simulink model "FOC_DQ0"  (R2022b)
settings: Solver=FixedStepAuto  StartTime=0.0  StopTime=20
values from neighbouring files (symbols this model uses):
  battery = struct()    [FOC_DQ0_parameters.m]
  motor = struct()    [FOC_DQ0_parameters.m]
libraries: simulink_extras x3, simulink x1
settings Model: Creator=dwegg  LastModifiedBy=dwegg
settings SolverCC: MaxConsecutiveZCs=auto  AlgebraicLoopSolver=TrustRegion
settings OptimizationCC: OptimizeBlockIOStorage=off  OptimizeDataStoreBuffers=off  BusAssignmentInplaceUpdate=off
settings DebuggingCC: UnconnectedInputMsg=warning  UnconnectedOutputMsg=warning  UnconnectedLineMsg=warning  SFUnexpectedBacktrackingDiag=warning  SFNoUnconditionalDefaultTransitionDiag=warning  SFMachineParentedDataDiag=warning
settings ModelReferenceCC: EnableRefExpFcnMdlSchedulingChecks=on
settings RTWCC: GenCodeOnly=on  GenerateReport=on  BuildConfiguration=Debug  LaunchReport=on  DLArmComputeVersion=19.05
settings CodeAppCC: ForceParamTrailComments=on  MATLABSourceComments=on  EnableCustomComments=on
settings GRTTargetCC: CombineSignalStateStructs=on  SupportVariableSizeSignals=on  MultiInstanceErrorCode=Warning

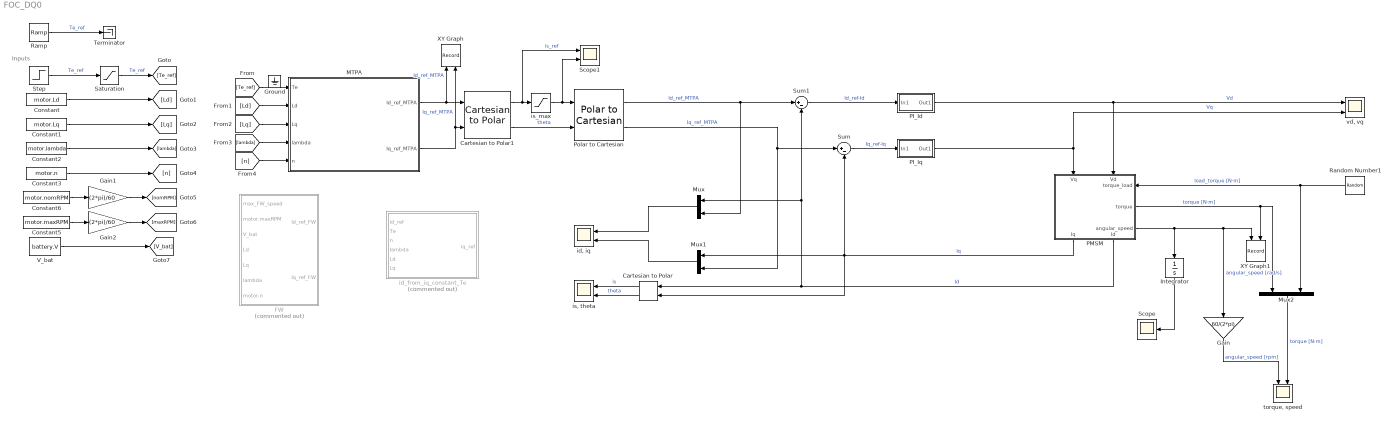
== system FOC_DQ0 ==
  note: Inputs
  Cartesian to Polar : simulink_extras/Transformations/Cartesian to Polar
  Cartesian to Polar1 : simulink_extras/Transformations/Cartesian to Polar
  Constant : Constant  Value=motor.Ld
  Constant1 : Constant  Value=motor.Lq
  Constant2 : Constant  Value=motor.lambda
  Constant3 : Constant  Value=motor.n
  Constant5 : Constant  Value=motor.maxRPM
  Constant6 : Constant  Value=motor.nomRPM
  FW : Subsystem  Commented=on
  Gain : Gain  Gain=60/(2*pi)
  Gain1 : Gain  Gain=(2*pi)/60
  Gain2 : Gain  Gain=(2*pi)/60
  Integrator : Integrator  UpperSaturationLimit=2*pi  LowerSaturationLimit=0  WrapState=on
  MTPA : Subsystem
  Mux : Mux  Inputs=2
  Mux1 : Mux  Inputs=2
  Mux2 : Mux  Inputs=2
  PI_Id : Subsystem
  PI_Iq : Subsystem
  PMSM : Subsystem
      settings: PortSchema="{\"entries\":[{\"content\":{\"sides\":[{\"content\":{\"connectorIds\":[\"In1\",\"In2\"]},\"type\":\"ConnectorPlacement.EquallySpacedRectSide\",\"uuid\":\"acf6d0e8-5fcc-4ac9-9f91-0b0686f5c890\"},{\"content\":{\"connectorIds\":[\"Out1\",\"Out2\"],\"side\":\"RIGHT\"},\"type\":\"ConnectorPlacement.EquallySpacedRectSide\",\"uuid\":\"62f3436c-1459-412f-a025-ace7c361d3d0\"},{\"content\":{\"connectorIds\":[\"In3\",\"Out3\",\"Out4\"],\"side\":\"TOP\"},\"type\":\"ConnectorPlacement.EquallySpacedRectSide\",\"uuid\":\"813607d4-1b75-442b-b64c-87c67b317e31\"},{\"content\":{\"connectorIds\":[],\"side\":\"HIDDEN\"},\"type\":\"ConnectorPlacement.EquallySpacedRectSide\",\"uuid\":\"b791fad5-6496-44b1-9d55-edef34be28ea\"}]},\"type\":\"ConnectorPlacement.EquallySpacedConnector\",\"uuid\":\"ea6ad5c4-a0c3-44bf-8a7e-ca4afd038dbb\"}],\"packageUris\":[\"http://schema.mathworks.com/mf0/Connector/R2020b\"],\"version\":\"1.0\"}"
      mask Display: image('$imagefile'); % Use "Edit Image" on toolstrip to change.
  Polar to Cartesian : simulink_extras/Transformations/Polar to Cartesian
  Ramp : simulink/Sources/Ramp  slope=-5  start=1  InitialOutput=40
  Random Number1 : RandomNumber  Variance=0  SampleTime=0.1
  Saturation : Saturate  UpperLimit=40  LowerLimit=-40
  Scope : Scope
  Scope1 : Scope  NumInputPorts=2
  Step : Step  After=26  SampleTime=0
  Sum : Sum  Inputs=|+-
  Sum1 : Sum  Inputs=|+-
  Terminator : Terminator
  V_bat : Constant  Value=battery.V
  XY Graph : Record  FileSettingsInternal="{\"entries\":[{\"content\":{\"excelSettings\":{\"content\":{},\"type\":\"Streamout.ExcelSettings\"}},\"type\":\"Streamout.FileSettingStorage\",\"uuid\":\"a65b38da-4a6e-42be-b919-12943431f1e8\"}],\"packageUris\":[\"http://schema.mathworks.com/mf0/streamout_blocks/R2020a\"],\"version\":\"1.0\"}"  Layout=[1 1]  SignalsInternal="{\"entries\":[{\"content\":{\"signals\":[{\"content\":{\"blockPath\":[\"FOC_DQ0/XY Graph\"],\"channel\":[],\"dimensions\":[1],\"domain\":\"FOC_DQ0/XY Graph\",\"lineColor\":\"#b746ff\",\"plots\":[1],\"port\":1,\"sid\":[\"\"],\"signalID\":27,\"signalName\":\"Id_ref_MTPA\"},\"type\":\"RecordBlkView.Signal\",\"uuid\":\"71ded6d7-b5de-456d-a39b-39459f0f97cd\"},{\"content\":{\"blockPath\":[\"FOC_DQ0/XY Graph\"],\"channel\":[],\"dimensions\":[1],\"domain\":\"FOC_DQ0/XY Graph\",\"lineColor\":\"#ff13a6\",\"plots\":[1],\"port\":2,\"sid\":[\"\"],\"signalID\":31,\"signalName\":\"Iq_ref_MTPA\"},\"type\":\"RecordBlkView.Signal\",\"uuid\":\"91d96bc1-a89e-499f-a0a8-186399ce3372\"}]},\"type\":\"RecordBlkView.InputSignals\",\"uuid\":\"76abfc2d-da4e-48c8-a2e1-e55e58ffb88b\"}],\"packageUris\":[\"http://schema.mathworks.com/mf0/streamout_blocks/R2020a\"],\"version\":\"1.0\"}"  VisualizationBindings="{\"xyplotplugin\":{\"info\":[{\"series\":[{\"bindingParametersList\":[{\"parameter\":\"X-Axis\",\"signalID\":27,\"signalName\":\"Id_ref_MTPA\"},{\"parameter\":\"Y-Axis\",\"signalID\":31,\"signalName\":\"Iq_ref_MTPA\"}],\"seriesID\":34336}],\"subplotID\":1}]}}"  CompatibilityTag=XY
  XY Graph1 : Record  FileSettingsInternal="{\"entries\":[{\"content\":{\"excelSettings\":{\"content\":{},\"type\":\"Streamout.ExcelSettings\"}},\"type\":\"Streamout.FileSettingStorage\",\"uuid\":\"c1a863bd-84bc-484d-b47a-9520c9f9713e\"}],\"packageUris\":[\"http://schema.mathworks.com/mf0/streamout_blocks/R2020a\"],\"version\":\"1.0\"}"  Layout=[1 1]  SignalsInternal="{\"entries\":[{\"content\":{\"signals\":[{\"content\":{\"blockPath\":[\"FOC_DQ0/XY Graph1\"],\"channel\":[],\"dimensions\":[1],\"domain\":\"FOC_DQ0/XY Graph1\",\"lineColor\":\"#a2142f\",\"plots\":[1],\"port\":1,\"sid\":[\"\"],\"signalID\":35,\"signalName\":\"angular_speed [rad/s]\"},\"type\":\"RecordBlkView.Signal\",\"uuid\":\"696599aa-ddef-40f7-9026-a933a86ecc6f\"},{\"content\":{\"blockPath\":[\"FOC_DQ0/XY Graph1\"],\"channel\":[],\"dimensions\":[1],\"domain\":\"FOC_DQ0/XY Graph1\",\"lineColor\":\"#139fff\",\"plots\":[1],\"port\":2,\"sid\":[\"\"],\"signalID\":39,\"signalName\":\"torque [N·m]\"},\"type\":\"RecordBlkView.Signal\",\"uuid\":\"06b63f20-2c7a-4cdb-9373-f78a38729ebe\"}]},\"type\":\"RecordBlkView.InputSignals\",\"uuid\":\"cbe1f972-30dc-467d-b6c0-ab8105ad27ef\"}],\"packageUris\":[\"http://schema.mathworks.com/mf0/streamout_blocks/R2020a\"],\"version\":\"1.0\"}"  VisualizationBindings="{\"xyplotplugin\":{\"info\":[{\"series\":[{\"bindingParametersList\":[{\"parameter\":\"X-Axis\",\"signalID\":35,\"signalName\":\"angular_speed [rad\\/s]\"},{\"parameter\":\"Y-Axis\",\"signalID\":39,\"signalName\":\"torque [N·m]\"}],\"seriesID\":51202}],\"subplotID\":1}]}}"  CompatibilityTag=XY
  "id, iq" : Scope  NumInputPorts=2
  id_from_iq_constant_Te : MATLAB Function  Commented=on  TreatAsAtomicUnit=on
  "is, theta" : Scope  NumInputPorts=2
  is_max : Saturate  UpperLimit=motor.I_max  LowerLimit=-motor.I_max
  "torque, speed" : Scope  NumInputPorts=2
  "vd, vq" : Scope  NumInputPorts=2
  Ground : Ground  IOType=siggen
  wires:
  Random Number1/1 -> Mux2/2, PMSM/3(torque_load)  "load_torque [N·m]"
  PI_Iq/1(Out1) -> "vd, vq"/2, PMSM/2(Vq)  "Vq"
  PI_Id/1(Out1) -> PMSM/1(Vd), "vd, vq"/1  "Vd"
  Sum/1 -> PI_Iq/1(In1)  "Iq_ref-Iq"
  Sum1/1 -> PI_Id/1(In1)  "Id_ref-Id"
  PMSM/1(Id) -> Mux/1, Sum1/2, Cartesian to Polar/1  "Id"
  Mux/1 -> "id, iq"/1
  Mux1/1 -> "id, iq"/2
  PMSM/3(torque) -> XY Graph1/2, Mux2/1  "torque [N·m]"
  PMSM/4(angular_speed) -> Integrator/1, XY Graph1/1, Gain/1  "angular_speed [rad/s]"
  Gain/1 -> "torque, speed"/1  "angular_speed [rpm]"
  Mux2/1 -> "torque, speed"/2  "torque [N·m]"
  Saturation/1 -> [Te_ref]  "Te_ref"
  Polar to Cartesian/1 -> Mux/2, Sum1/1  "Id_ref_MTPA"
  Polar to Cartesian/2 -> Sum/1, Mux1/2  "Iq_ref_MTPA"
  Constant6/1 -> Gain1/1
  Cartesian to Polar/1 -> "is, theta"/1  "is"
  Cartesian to Polar/2 -> "is, theta"/2  "theta"
  Constant/1 -> [Ld]
  Constant1/1 -> [Lq]
  Constant2/1 -> [lambda]
  Constant3/1 -> [n]
  Gain1/1 -> [nomRPM]
  Constant5/1 -> Gain2/1
  Gain2/1 -> [maxRPM]
  V_bat/1 -> [V_bat]
  [Te_ref] -> MTPA/1(Te)
  [Ld] -> MTPA/2(Ld)
  [Lq] -> MTPA/3(Lq)
  [lambda] -> MTPA/4(lambda)
  [n] -> MTPA/5(n)
  Step/1 -> Saturation/1  "Te_ref"
  MTPA/1(Id_ref_MTPA) -> XY Graph/1, Cartesian to Polar1/1  "Id_ref_MTPA"
  MTPA/2(Iq_ref_MTPA) -> XY Graph/2, Cartesian to Polar1/2  "Iq_ref_MTPA"
  Cartesian to Polar1/2 -> Polar to Cartesian/2  "theta"
  Cartesian to Polar1/1 -> Scope1/1, is_max/1  "is_ref"
  is_max/1 -> Scope1/2, Polar to Cartesian/1
  PMSM/2(Iq) -> Mux1/1, Cartesian to Polar/2, Sum/2  "Iq"
  Integrator/1 -> Scope/1
  Ramp/1 -> Terminator/1  "Te_ref"

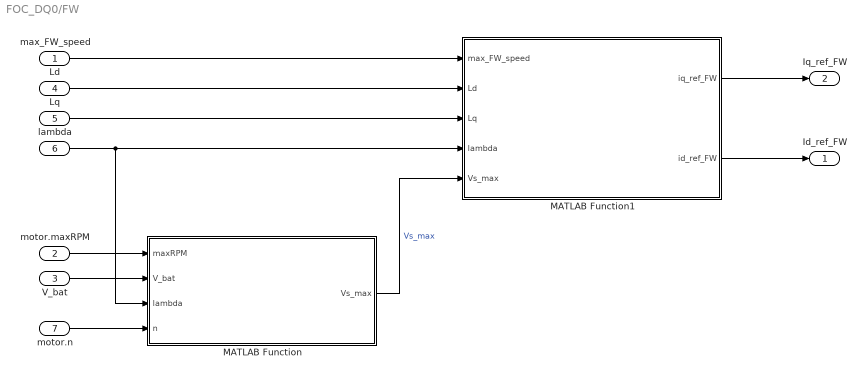
== system FOC_DQ0/FW ==
  max_FW_speed : Inport
  motor.maxRPM : Inport  Port=2
  V_bat : Inport  Port=3
  Ld : Inport  Port=4
  Lq : Inport  Port=5
  lambda : Inport  Port=6
  motor.n : Inport  Port=7
  MATLAB Function : MATLAB Function  TreatAsAtomicUnit=on
  MATLAB Function1 : MATLAB Function  TreatAsAtomicUnit=on
  Id_ref_FW : Outport
  Iq_ref_FW : Outport  Port=2
  wires:
  motor.maxRPM/1 -> MATLAB Function/1(maxRPM)
  V_bat/1 -> MATLAB Function/2(V_bat)
  MATLAB Function/1(Vs_max) -> MATLAB Function1/5(Vs_max)  "Vs_max"
  max_FW_speed/1 -> MATLAB Function1/1(max_FW_speed)
  Ld/1 -> MATLAB Function1/2(Ld)
  Lq/1 -> MATLAB Function1/3(Lq)
  lambda/1 -> MATLAB Function/3(lambda), MATLAB Function1/4(lambda)
  MATLAB Function1/1(iq_ref_FW) -> Iq_ref_FW/1
  MATLAB Function1/2(id_ref_FW) -> Id_ref_FW/1
  motor.n/1 -> MATLAB Function/4(n)

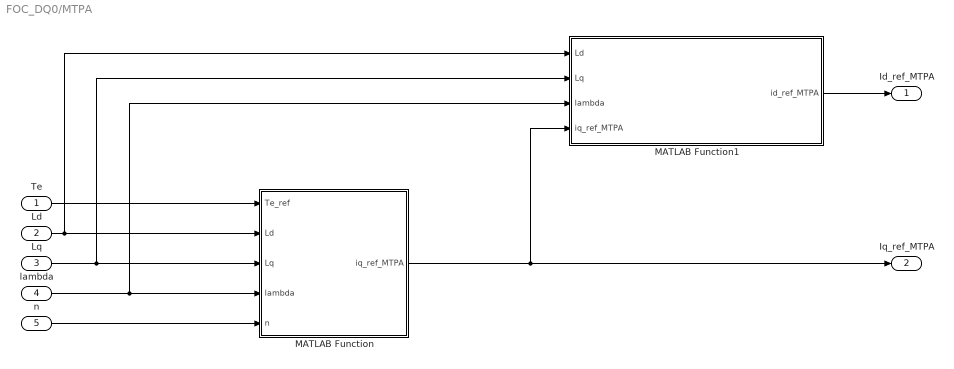
== system FOC_DQ0/MTPA ==
  Te : Inport
  Ld : Inport  Port=2
  Lq : Inport  Port=3
  lambda : Inport  Port=4
  n : Inport  Port=5
  MATLAB Function : MATLAB Function  TreatAsAtomicUnit=on
  MATLAB Function1 : MATLAB Function  TreatAsAtomicUnit=on
  Id_ref_MTPA : Outport
  Iq_ref_MTPA : Outport  Port=2
  wires:
  MATLAB Function/1(iq_ref_MTPA) -> MATLAB Function1/4(iq_ref_MTPA), Iq_ref_MTPA/1
  Te/1 -> MATLAB Function/1(Te_ref)
  Ld/1 -> MATLAB Function/2(Ld), MATLAB Function1/1(Ld)
  Lq/1 -> MATLAB Function1/2(Lq), MATLAB Function/3(Lq)
  lambda/1 -> MATLAB Function1/3(lambda), MATLAB Function/4(lambda)
  n/1 -> MATLAB Function/5(n)
  MATLAB Function1/1(id_ref_MTPA) -> Id_ref_MTPA/1

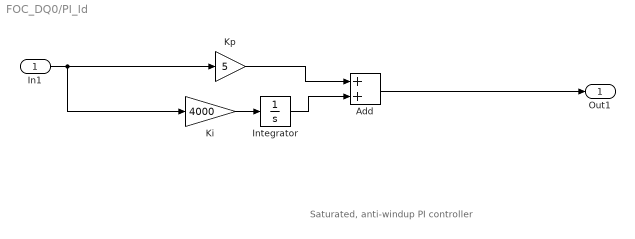
== system FOC_DQ0/PI_Id ==
  note: Saturated, anti-windup PI controller
  In1 : Inport
  Add : Sum
  Integrator : Integrator
  Ki : Gain  Gain=4000
  Kp : Gain  Gain=5
  Out1 : Outport
  wires:
  In1/1 -> Ki/1, Kp/1
  Kp/1 -> Add/1
  Integrator/1 -> Add/2
  Ki/1 -> Integrator/1
  Add/1 -> Out1/1

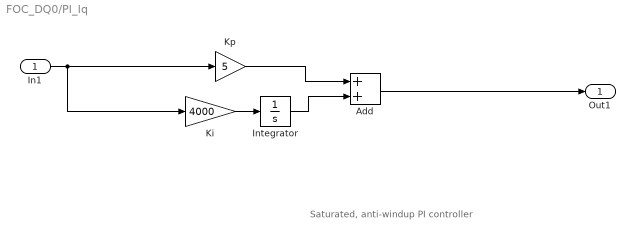
== system FOC_DQ0/PI_Iq ==
  note: Saturated, anti-windup PI controller
  In1 : Inport
  Add : Sum
  Integrator : Integrator
  Ki : Gain  Gain=4000
  Kp : Gain  Gain=5
  Out1 : Outport
  wires:
  Ki/1 -> Integrator/1
  Integrator/1 -> Add/2
  Kp/1 -> Add/1
  Add/1 -> Out1/1
  In1/1 -> Ki/1, Kp/1

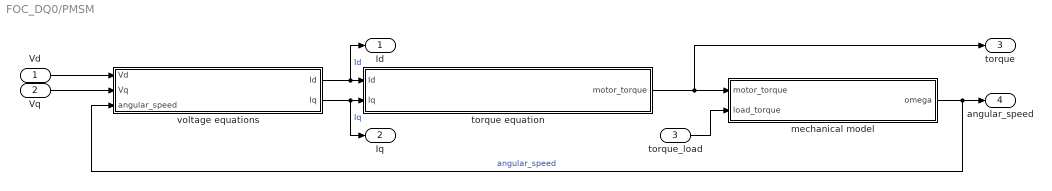
== system FOC_DQ0/PMSM ==
  Vd : Inport
  Vq : Inport  Port=2
  torque_load : Inport  Port=3
  mechanical model : Subsystem
      mask Display: image('$imagefile'); % Use "Edit Image" on toolstrip to change.
  torque equation : Subsystem
      mask Display: image('$imagefile'); % Use "Edit Image" on toolstrip to change.
  voltage equations : Subsystem
      mask Display: image('$imagefile'); % Use "Edit Image" on toolstrip to change.
  Id : Outport
  Iq : Outport  Port=2
  torque : Outport  Port=3
  angular_speed : Outport  Port=4
  wires:
  torque equation/1(motor_torque) -> torque/1, mechanical model/1(motor_torque)
  torque_load/1 -> mechanical model/2(load_torque)
  mechanical model/1(omega) -> angular_speed/1, voltage equations/3(angular_speed)  "angular_speed"
  voltage equations/2(Iq) -> Iq/1, torque equation/2(Iq)  "Iq"
  voltage equations/1(Id) -> Id/1, torque equation/1(Id)  "Id"
  Vd/1 -> voltage equations/1(Vd)
  Vq/1 -> voltage equations/2(Vq)

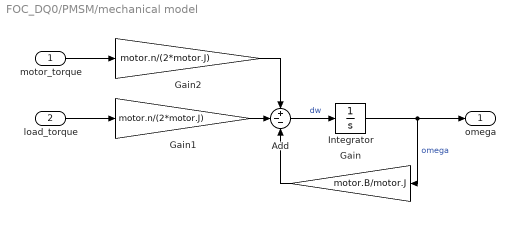
== system FOC_DQ0/PMSM/mechanical model ==
  motor_torque : Inport
  load_torque : Inport  Port=2
  Add : Sum  Inputs=+--
  Gain : Gain  Gain=motor.B/motor.J
  Gain1 : Gain  Gain=motor.n/(2*motor.J)
  Gain2 : Gain  Gain=motor.n/(2*motor.J)
  Integrator : Integrator
  omega : Outport
  wires:
  Gain1/1 -> Add/2
  Gain/1 -> Add/3
  Gain2/1 -> Add/1
  Add/1 -> Integrator/1  "dw"
  Integrator/1 -> omega/1, Gain/1  "omega"
  motor_torque/1 -> Gain2/1
  load_torque/1 -> Gain1/1

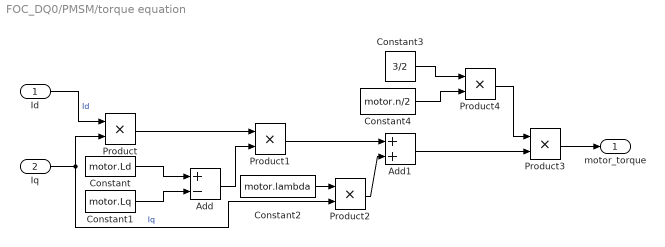
== system FOC_DQ0/PMSM/torque equation ==
  Id : Inport
  Iq : Inport  Port=2
  Add : Sum  Inputs=+-
  Add1 : Sum
  Constant : Constant  Value=motor.Ld
  Constant1 : Constant  Value=motor.Lq
  Constant2 : Constant  Value=motor.lambda
  Constant3 : Constant  Value=3/2
  Constant4 : Constant  Value=motor.n/2
  Product{,1..4} (5 alike) : Product
  motor_torque : Outport
  wires:
  Product1/1 -> Add1/1
  Add/1 -> Product1/2
  Constant4/1 -> Product4/2
  Constant2/1 -> Product2/1
  Add1/1 -> Product3/2
  Constant/1 -> Add/1
  Product/1 -> Product1/1
  Product4/1 -> Product3/1
  Constant3/1 -> Product4/1
  Product2/1 -> Add1/2
  Iq/1 -> Product/2, Product2/2  "Iq"
  Constant1/1 -> Add/2
  Product3/1 -> motor_torque/1
  Id/1 -> Product/1  "Id"

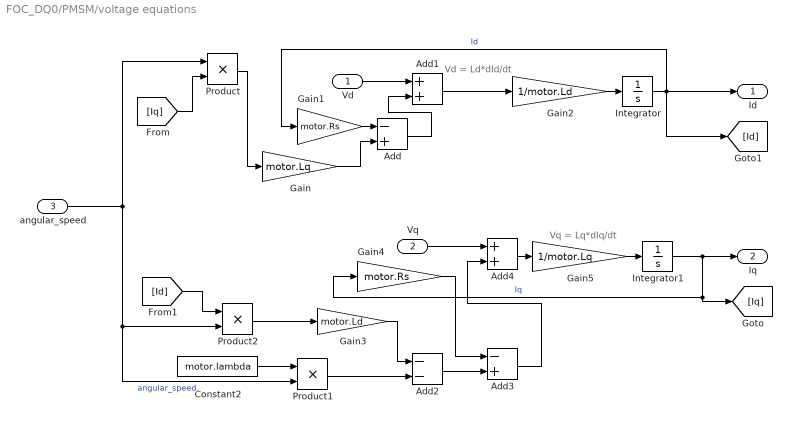
== system FOC_DQ0/PMSM/voltage equations ==
  note: Vd = Ld*dId/dt
  note: Vq = Lq*dIq/dt
  Vd : Inport
  Vq : Inport  Port=2
  angular_speed : Inport  Port=3
  Add : Sum  Inputs=-+
  Add1 : Sum
  Add2 : Sum  Inputs=--
  Add3 : Sum  Inputs=-+
  Add4 : Sum
  Constant2 : Constant  Value=motor.lambda
  Gain : Gain  Gain=motor.Lq
  Gain1 : Gain  Gain=motor.Rs
  Gain2 : Gain  Gain=1/motor.Ld
  Gain3 : Gain  Gain=motor.Ld
  Gain4 : Gain  Gain=motor.Rs
  Gain5 : Gain  Gain=1/motor.Lq
  Integrator : Integrator
  Integrator1 : Integrator
  Product : Product
  Product1 : Product
  Product2 : Product
  Id : Outport
  Iq : Outport  Port=2
  wires:
  angular_speed/1 -> Product2/2, Product1/2, Product/1  "angular_speed"
  Product/1 -> Gain/1
  Gain/1 -> Add/2
  Gain1/1 -> Add/1
  Integrator/1 -> Gain1/1, [Id], Id/1  "Id"
  Gain2/1 -> Integrator/1
  Add1/1 -> Gain2/1
  Add/1 -> Add1/2
  Vd/1 -> Add1/1
  Constant2/1 -> Product1/1
  Product2/1 -> Gain3/1
  Gain3/1 -> Add2/1
  Product1/1 -> Add2/2
  Add2/1 -> Add3/2
  Gain4/1 -> Add3/1
  Add3/1 -> Add4/2
  Vq/1 -> Add4/1
  Add4/1 -> Gain5/1
  Gain5/1 -> Integrator1/1
  [Iq] -> Product/2
  [Id] -> Product2/1
  Integrator1/1 -> [Iq], Gain4/1, Iq/1  "Iq"

== matlab function FOC_DQ0/MTPA/MATLAB Function1 ==
  data: Ld input; id_ref_MTPA output; Lq input; lambda input; iq_ref_MTPA input
function id_ref_MTPA = id_ref_MTPA_from_iq_ref_MTPA(Ld, Lq, lambda, iq_ref_MTPA)
    id_ref_MTPA = -lambda/(2*(Ld-Lq)) - sqrt((lambda/(2*(Ld-Lq)))^2+iq_ref_MTPA.^2);
end

== matlab function FOC_DQ0/MTPA/MATLAB Function ==
  data: Te_ref input; iq_ref_MTPA output; Ld input; Lq input; lambda input; n input
function iq_ref_MTPA = iq_ref_MTPA_from_Te_ref(Te_ref, Ld, Lq, lambda, n)
% solve iq^4 + iq*Te*lambda/((3/2)*(n/2)*(Ld-Lq)^2) - Te^2/(((3/2)*(n/2)*(Ld-Lq))^2) = 0 for iq
    f = @(iq) iq^4 + iq*Te_ref*lambda/((3/2)*(n/2)*(Ld-Lq)^2) - Te_ref^2/(((3/2)*(n/2)*(Ld-Lq))^2);

    % Use fzero to solve for iq
    iq_ref_MTPA = fzero(f, 0);
end

== matlab function FOC_DQ0/FW/MATLAB Function ==
  data: maxRPM input; Vs_max output; V_bat input; lambda input; n input
function Vs_max = Vs_max_from_maxRPM_V_bat(maxRPM, V_bat, lambda, n)
    V_b = lambda * maxRPM*(2*pi/60) / (n/2); % [V] Base voltage
    Vs_max = V_bat / (sqrt(3)*V_b);

== matlab function FOC_DQ0/FW/MATLAB Function1 ==
  data: max_FW_speed input; Ld input; Lq input; iq_ref_FW output; id_ref_FW output; lambda input; Vs_max input
function [iq_ref_FW, id_ref_FW] = fcn(max_FW_speed, Ld, Lq, lambda, Vs_max)
    h_ellipse = -lambda/Ld;
    a_ellipse = Vs_max./(Ld.*max_FW_speed);
    b_ellipse = Vs_max./(Lq.*max_FW_speed);
    
    t=-pi:0.01:pi;
    
    id_ref_FW=h_ellipse+a_ellipse.*cos(t);
    iq_ref_FW=b_ellipse.*sin(t);

== matlab function FOC_DQ0/id_from_iq_constant_Te ==
  data: id_ref input; iq_ref output; Te input; n input; lambda input; Ld input; Lq input
function iq_ref = id_from_iq_constantTe(id_ref, Te, n, lambda, Ld, Lq)
iq_ref = 4*Te/(3*n*(lambda+(Ld-Lq)*id_ref));
